simulink model "c00007M_harness"  (R2018a)
settings: Solver=ode3  StartTime=0.0  StopTime=10.0  RelTol=1e-3  EnableMultiTasking=on
undefined symbols (not defined in the file): b, DiscIntNeverNeededParam, J, K, L, PosMinimaW3, PosMinimaW4, R, sigbuilder_block
(part 6 of 74)

== system c00007M_harness/Eval92 ==
  In1 : Inport
  In2 : Inport  Port=2
  In3 : Inport  Port=3
  In4 : Inport  Port=4
  Data Type Conversion{,1..3} (4 alike) : DataTypeConversion
  Memory{1..4} (4 alike) : Memory  InitialCondition=1
  MinMax : MinMax  Inputs=4
  MinMax{1..4} (4 alike) : MinMax  Inputs=2
  ROOut{1..4} (4 alike) : RelationalOperator  Operator===  OutDataTypeStr=boolean  RndMeth=Simplest
  Out1 : Outport
  wires:
  Data Type Conversion3/1 -> MinMax4/1
  Data Type Conversion2/1 -> MinMax3/1
  Data Type Conversion1/1 -> MinMax2/1
  Data Type Conversion/1 -> MinMax1/1
  MinMax1/1 -> Memory1/1, MinMax/1
  ROOut4/1 -> Data Type Conversion3/1
  MinMax2/1 -> Memory2/1, MinMax/2
  ROOut1/1 -> Data Type Conversion/1
  Memory2/1 -> MinMax2/2
  Memory4/1 -> MinMax4/2
  Memory3/1 -> MinMax3/2
  ROOut2/1 -> Data Type Conversion1/1
  ROOut3/1 -> Data Type Conversion2/1
  MinMax3/1 -> Memory3/1, MinMax/3
  MinMax4/1 -> Memory4/1, MinMax/4
  Memory1/1 -> MinMax1/2
  [out4] -> ROOut4/2
  In4/1 -> ROOut4/1
  [out2] -> ROOut2/2
  In1/1 -> ROOut1/1
  In2/1 -> ROOut2/1
  [out1] -> ROOut1/2
  In3/1 -> ROOut3/1
  [out3] -> ROOut3/2
  MinMax/1 -> Out1/1

== system c00007M_harness/Eval93 ==
  In1 : Inport
  In2 : Inport  Port=2
  In3 : Inport  Port=3
  In4 : Inport  Port=4
  Data Type Conversion{,1..3} (4 alike) : DataTypeConversion
  Memory{1..4} (4 alike) : Memory  InitialCondition=1
  MinMax : MinMax  Inputs=4
  MinMax{1..4} (4 alike) : MinMax  Inputs=2
  ROOut{1..4} (4 alike) : RelationalOperator  Operator===  OutDataTypeStr=boolean  RndMeth=Simplest
  Out1 : Outport
  wires:
  Data Type Conversion3/1 -> MinMax4/1
  Data Type Conversion2/1 -> MinMax3/1
  Data Type Conversion1/1 -> MinMax2/1
  Data Type Conversion/1 -> MinMax1/1
  MinMax1/1 -> Memory1/1, MinMax/1
  ROOut4/1 -> Data Type Conversion3/1
  MinMax2/1 -> Memory2/1, MinMax/2
  ROOut1/1 -> Data Type Conversion/1
  Memory2/1 -> MinMax2/2
  Memory4/1 -> MinMax4/2
  Memory3/1 -> MinMax3/2
  ROOut2/1 -> Data Type Conversion1/1
  ROOut3/1 -> Data Type Conversion2/1
  MinMax3/1 -> Memory3/1, MinMax/3
  MinMax4/1 -> Memory4/1, MinMax/4
  Memory1/1 -> MinMax1/2
  [out4] -> ROOut4/2
  In4/1 -> ROOut4/1
  [out2] -> ROOut2/2
  In1/1 -> ROOut1/1
  In2/1 -> ROOut2/1
  [out1] -> ROOut1/2
  In3/1 -> ROOut3/1
  [out3] -> ROOut3/2
  MinMax/1 -> Out1/1

== system c00007M_harness/Eval94 ==
  In1 : Inport
  In2 : Inport  Port=2
  In3 : Inport  Port=3
  In4 : Inport  Port=4
  Data Type Conversion{,1..3} (4 alike) : DataTypeConversion
  Memory{1..4} (4 alike) : Memory  InitialCondition=1
  MinMax : MinMax  Inputs=4
  MinMax{1..4} (4 alike) : MinMax  Inputs=2
  ROOut{1..4} (4 alike) : RelationalOperator  Operator===  OutDataTypeStr=boolean  RndMeth=Simplest
  Out1 : Outport
  wires:
  Data Type Conversion3/1 -> MinMax4/1
  Data Type Conversion2/1 -> MinMax3/1
  Data Type Conversion1/1 -> MinMax2/1
  Data Type Conversion/1 -> MinMax1/1
  MinMax1/1 -> Memory1/1, MinMax/1
  ROOut4/1 -> Data Type Conversion3/1
  MinMax2/1 -> Memory2/1, MinMax/2
  ROOut1/1 -> Data Type Conversion/1
  Memory2/1 -> MinMax2/2
  Memory4/1 -> MinMax4/2
  Memory3/1 -> MinMax3/2
  ROOut2/1 -> Data Type Conversion1/1
  ROOut3/1 -> Data Type Conversion2/1
  MinMax3/1 -> Memory3/1, MinMax/3
  MinMax4/1 -> Memory4/1, MinMax/4
  Memory1/1 -> MinMax1/2
  [out4] -> ROOut4/2
  In4/1 -> ROOut4/1
  [out2] -> ROOut2/2
  In1/1 -> ROOut1/1
  In2/1 -> ROOut2/1
  [out1] -> ROOut1/2
  In3/1 -> ROOut3/1
  [out3] -> ROOut3/2
  MinMax/1 -> Out1/1

== system c00007M_harness/Eval95 ==
  In1 : Inport
  In2 : Inport  Port=2
  In3 : Inport  Port=3
  In4 : Inport  Port=4
  Data Type Conversion{,1..3} (4 alike) : DataTypeConversion
  Memory{1..4} (4 alike) : Memory  InitialCondition=1
  MinMax : MinMax  Inputs=4
  MinMax{1..4} (4 alike) : MinMax  Inputs=2
  ROOut{1..4} (4 alike) : RelationalOperator  Operator===  OutDataTypeStr=boolean  RndMeth=Simplest
  Out1 : Outport
  wires:
  Data Type Conversion3/1 -> MinMax4/1
  Data Type Conversion2/1 -> MinMax3/1
  Data Type Conversion1/1 -> MinMax2/1
  Data Type Conversion/1 -> MinMax1/1
  MinMax1/1 -> Memory1/1, MinMax/1
  ROOut4/1 -> Data Type Conversion3/1
  MinMax2/1 -> Memory2/1, MinMax/2
  ROOut1/1 -> Data Type Conversion/1
  Memory2/1 -> MinMax2/2
  Memory4/1 -> MinMax4/2
  Memory3/1 -> MinMax3/2
  ROOut2/1 -> Data Type Conversion1/1
  ROOut3/1 -> Data Type Conversion2/1
  MinMax3/1 -> Memory3/1, MinMax/3
  MinMax4/1 -> Memory4/1, MinMax/4
  Memory1/1 -> MinMax1/2
  [out4] -> ROOut4/2
  In4/1 -> ROOut4/1
  [out2] -> ROOut2/2
  In1/1 -> ROOut1/1
  In2/1 -> ROOut2/1
  [out1] -> ROOut1/2
  In3/1 -> ROOut3/1
  [out3] -> ROOut3/2
  MinMax/1 -> Out1/1

== system c00007M_harness/Eval96 ==
  In1 : Inport
  In2 : Inport  Port=2
  In3 : Inport  Port=3
  In4 : Inport  Port=4
  Data Type Conversion{,1..3} (4 alike) : DataTypeConversion
  Memory{1..4} (4 alike) : Memory  InitialCondition=1
  MinMax : MinMax  Inputs=4
  MinMax{1..4} (4 alike) : MinMax  Inputs=2
  ROOut{1..4} (4 alike) : RelationalOperator  Operator===  OutDataTypeStr=boolean  RndMeth=Simplest
  Out1 : Outport
  wires:
  Data Type Conversion3/1 -> MinMax4/1
  Data Type Conversion2/1 -> MinMax3/1
  Data Type Conversion1/1 -> MinMax2/1
  Data Type Conversion/1 -> MinMax1/1
  MinMax1/1 -> Memory1/1, MinMax/1
  ROOut4/1 -> Data Type Conversion3/1
  MinMax2/1 -> Memory2/1, MinMax/2
  ROOut1/1 -> Data Type Conversion/1
  Memory2/1 -> MinMax2/2
  Memory4/1 -> MinMax4/2
  Memory3/1 -> MinMax3/2
  ROOut2/1 -> Data Type Conversion1/1
  ROOut3/1 -> Data Type Conversion2/1
  MinMax3/1 -> Memory3/1, MinMax/3
  MinMax4/1 -> Memory4/1, MinMax/4
  Memory1/1 -> MinMax1/2
  [out4] -> ROOut4/2
  In4/1 -> ROOut4/1
  [out2] -> ROOut2/2
  In1/1 -> ROOut1/1
  In2/1 -> ROOut2/1
  [out1] -> ROOut1/2
  In3/1 -> ROOut3/1
  [out3] -> ROOut3/2
  MinMax/1 -> Out1/1

== system c00007M_harness/Eval97 ==
  In1 : Inport
  In2 : Inport  Port=2
  In3 : Inport  Port=3
  In4 : Inport  Port=4
  Data Type Conversion{,1..3} (4 alike) : DataTypeConversion
  Memory{1..4} (4 alike) : Memory  InitialCondition=1
  MinMax : MinMax  Inputs=4
  MinMax{1..4} (4 alike) : MinMax  Inputs=2
  ROOut{1..4} (4 alike) : RelationalOperator  Operator===  OutDataTypeStr=boolean  RndMeth=Simplest
  Out1 : Outport
  wires:
  Data Type Conversion3/1 -> MinMax4/1
  Data Type Conversion2/1 -> MinMax3/1
  Data Type Conversion1/1 -> MinMax2/1
  Data Type Conversion/1 -> MinMax1/1
  MinMax1/1 -> Memory1/1, MinMax/1
  ROOut4/1 -> Data Type Conversion3/1
  MinMax2/1 -> Memory2/1, MinMax/2
  ROOut1/1 -> Data Type Conversion/1
  Memory2/1 -> MinMax2/2
  Memory4/1 -> MinMax4/2
  Memory3/1 -> MinMax3/2
  ROOut2/1 -> Data Type Conversion1/1
  ROOut3/1 -> Data Type Conversion2/1
  MinMax3/1 -> Memory3/1, MinMax/3
  MinMax4/1 -> Memory4/1, MinMax/4
  Memory1/1 -> MinMax1/2
  [out4] -> ROOut4/2
  In4/1 -> ROOut4/1
  [out2] -> ROOut2/2
  In1/1 -> ROOut1/1
  In2/1 -> ROOut2/1
  [out1] -> ROOut1/2
  In3/1 -> ROOut3/1
  [out3] -> ROOut3/2
  MinMax/1 -> Out1/1

== system c00007M_harness/Eval98 ==
  In1 : Inport
  In2 : Inport  Port=2
  In3 : Inport  Port=3
  In4 : Inport  Port=4
  Data Type Conversion{,1..3} (4 alike) : DataTypeConversion
  Memory{1..4} (4 alike) : Memory  InitialCondition=1
  MinMax : MinMax  Inputs=4
  MinMax{1..4} (4 alike) : MinMax  Inputs=2
  ROOut{1..4} (4 alike) : RelationalOperator  Operator===  OutDataTypeStr=boolean  RndMeth=Simplest
  Out1 : Outport
  wires:
  Data Type Conversion3/1 -> MinMax4/1
  Data Type Conversion2/1 -> MinMax3/1
  Data Type Conversion1/1 -> MinMax2/1
  Data Type Conversion/1 -> MinMax1/1
  MinMax1/1 -> Memory1/1, MinMax/1
  ROOut4/1 -> Data Type Conversion3/1
  MinMax2/1 -> Memory2/1, MinMax/2
  ROOut1/1 -> Data Type Conversion/1
  Memory2/1 -> MinMax2/2
  Memory4/1 -> MinMax4/2
  Memory3/1 -> MinMax3/2
  ROOut2/1 -> Data Type Conversion1/1
  ROOut3/1 -> Data Type Conversion2/1
  MinMax3/1 -> Memory3/1, MinMax/3
  MinMax4/1 -> Memory4/1, MinMax/4
  Memory1/1 -> MinMax1/2
  [out4] -> ROOut4/2
  In4/1 -> ROOut4/1
  [out2] -> ROOut2/2
  In1/1 -> ROOut1/1
  In2/1 -> ROOut2/1
  [out1] -> ROOut1/2
  In3/1 -> ROOut3/1
  [out3] -> ROOut3/2
  MinMax/1 -> Out1/1

== system c00007M_harness/Eval99 ==
  In1 : Inport
  In2 : Inport  Port=2
  In3 : Inport  Port=3
  In4 : Inport  Port=4
  Data Type Conversion{,1..3} (4 alike) : DataTypeConversion
  Memory{1..4} (4 alike) : Memory  InitialCondition=1
  MinMax : MinMax  Inputs=4
  MinMax{1..4} (4 alike) : MinMax  Inputs=2
  ROOut{1..4} (4 alike) : RelationalOperator  Operator===  OutDataTypeStr=boolean  RndMeth=Simplest
  Out1 : Outport
  wires:
  Data Type Conversion3/1 -> MinMax4/1
  Data Type Conversion2/1 -> MinMax3/1
  Data Type Conversion1/1 -> MinMax2/1
  Data Type Conversion/1 -> MinMax1/1
  MinMax1/1 -> Memory1/1, MinMax/1
  ROOut4/1 -> Data Type Conversion3/1
  MinMax2/1 -> Memory2/1, MinMax/2
  ROOut1/1 -> Data Type Conversion/1
  Memory2/1 -> MinMax2/2
  Memory4/1 -> MinMax4/2
  Memory3/1 -> MinMax3/2
  ROOut2/1 -> Data Type Conversion1/1
  ROOut3/1 -> Data Type Conversion2/1
  MinMax3/1 -> Memory3/1, MinMax/3
  MinMax4/1 -> Memory4/1, MinMax/4
  Memory1/1 -> MinMax1/2
  [out4] -> ROOut4/2
  In4/1 -> ROOut4/1
  [out2] -> ROOut2/2
  In1/1 -> ROOut1/1
  In2/1 -> ROOut2/1
  [out1] -> ROOut1/2
  In3/1 -> ROOut3/1
  [out3] -> ROOut3/2
  MinMax/1 -> Out1/1

== system c00007M_harness/Inputs ==
  Demux : Demux  Tag=STV Demux  Outputs=14
  FromWs : FromWorkspace  Tag=STV FromWs  VariableName=tuvar  SampleTime=0
  DW1 : Outport  Tag=STV Outport
  DW2 : Outport  Tag=STV Outport  Port=2
  DW3 : Outport  Tag=STV Outport  Port=3
  P1W2 : Outport  Tag=STV Outport  Port=4
  P2W3 : Outport  Tag=STV Outport  Port=5
  P3W4 : Outport  Tag=STV Outport  Port=6
  O1 : Outport  Tag=STV Outport  Port=7
  O2 : Outport  Tag=STV Outport  Port=8
  O3 : Outport  Tag=STV Outport  Port=9
  O4 : Outport  Tag=STV Outport  Port=10
  LD : Outport  Tag=STV Outport  Port=11
  CW1C : Outport  Tag=STV Outport  Port=12
  CW2C : Outport  Tag=STV Outport  Port=13
  CW4C : Outport  Tag=STV Outport  Port=14
  wires:
  Demux/14 -> CW4C/1
  Demux/13 -> CW2C/1
  Demux/12 -> CW1C/1
  Demux/11 -> LD/1
  Demux/10 -> O4/1
  Demux/9 -> O3/1
  Demux/8 -> O2/1
  Demux/7 -> O1/1
  Demux/6 -> P3W4/1
  Demux/5 -> P2W3/1
  Demux/4 -> P1W2/1
  Demux/3 -> DW3/1
  Demux/2 -> DW2/1
  Demux/1 -> DW1/1
  FromWs/1 -> Demux/1

== system c00007M_harness/M001 ==
  DW1 : Inport  OutMin=0  OutMax=4  OutDataTypeStr=int8
  DW2 : Inport  Port=2  OutMin=0  OutMax=4  OutDataTypeStr=int8
  DW3 : Inport  Port=3  OutMin=0  OutMax=4  OutDataTypeStr=int8
  P1W2 : Inport  Port=4  OutMin=0  OutMax=4  OutDataTypeStr=int8
  P2W3 : Inport  Port=5  OutMin=0  OutMax=4  OutDataTypeStr=int8
  P3W4 : Inport  Port=6  OutMin=0  OutMax=4  OutDataTypeStr=int8
  O1 : Inport  Port=7  OutDataTypeStr=boolean
  O2 : Inport  Port=8  OutDataTypeStr=boolean
  O3 : Inport  Port=9  OutDataTypeStr=boolean
  O4 : Inport  Port=10  OutDataTypeStr=boolean
  LD : Inport  Port=11  OutDataTypeStr=boolean
  CW1C : Inport  Port=12  OutMin=0  OutMax=4  OutDataTypeStr=int8
  CW2C : Inport  Port=13  OutMin=0  OutMax=4  OutDataTypeStr=int8
  CW4C : Inport  Port=14  OutMin=0  OutMax=4  OutDataTypeStr=int8
  Cyber : Subsystem
  M{,1..3} (4 alike) : Memory
  Physical : Subsystem
  S1 : Subsystem
  S2 : Subsystem
  S3 : Subsystem
  S4 : Subsystem
  W1Pos : Outport
  W2Pos : Outport  Port=2
  W3Pos : Outport  Port=3
  W4Pos : Outport  Port=4
  wires:
  M3/1 -> Cyber/4(PosW4)
  P2W3/1 -> Cyber/9(P2W3)
  S1/1(SensorOut) -> M/1
  CW2C/1 -> Cyber/17(CW2C)
  CW4C/1 -> Cyber/18(CW4C)
  Physical/1(W1) -> W1Pos/1, S1/1(PhyMeasure)
  O4/1 -> Cyber/14(OW4)
  S3/1(SensorOut) -> M2/1
  O2/1 -> Cyber/12(OW2)
  Cyber/3(W3) -> Physical/3(InW3)
  LD/1 -> Cyber/15(LD)
  O1/1 -> Cyber/11(OW1)
  Cyber/1(W1) -> Physical/1(InW1)
  Cyber/2(W2) -> Physical/2(InW2)
  M2/1 -> Cyber/3(PosW3)
  P1W2/1 -> Cyber/8(P1W2)
  CW1C/1 -> Cyber/16(CW1C)
  O3/1 -> Cyber/13(OW3)
  DW3/1 -> Cyber/7(DW3)
  S4/1(SensorOut) -> M3/1
  M1/1 -> Cyber/2(PosW2)
  Physical/3(W3) -> W3Pos/1, S3/1(PhyMeasure)
  M/1 -> Cyber/1(PosW1)
  DW1/1 -> Cyber/5(DW1)
  Physical/2(W2) -> W2Pos/1, S2/1(PhyMeasure)
  S2/1(SensorOut) -> M1/1
  P3W4/1 -> Cyber/10(P3W4)
  DW2/1 -> Cyber/6(DW2)
  Physical/4(W4) -> W4Pos/1, S4/1(PhyMeasure)
  Cyber/4(W4) -> Physical/4(InW4)

== system c00007M_harness/M002 ==
  DW1 : Inport  OutMin=0  OutMax=4  OutDataTypeStr=int8
  DW2 : Inport  Port=2  OutMin=0  OutMax=4  OutDataTypeStr=int8
  DW3 : Inport  Port=3  OutMin=0  OutMax=4  OutDataTypeStr=int8
  P1W2 : Inport  Port=4  OutMin=0  OutMax=4  OutDataTypeStr=int8
  P2W3 : Inport  Port=5  OutMin=0  OutMax=4  OutDataTypeStr=int8
  P3W4 : Inport  Port=6  OutMin=0  OutMax=4  OutDataTypeStr=int8
  O1 : Inport  Port=7  OutDataTypeStr=boolean
  O2 : Inport  Port=8  OutDataTypeStr=boolean
  O3 : Inport  Port=9  OutDataTypeStr=boolean
  O4 : Inport  Port=10  OutDataTypeStr=boolean
  LD : Inport  Port=11  OutDataTypeStr=boolean
  CW1C : Inport  Port=12  OutMin=0  OutMax=4  OutDataTypeStr=int8
  CW2C : Inport  Port=13  OutMin=0  OutMax=4  OutDataTypeStr=int8
  CW4C : Inport  Port=14  OutMin=0  OutMax=4  OutDataTypeStr=int8
  Cyber : Subsystem
  M{,1..3} (4 alike) : Memory
  Physical : Subsystem
  S1 : Subsystem
  S2 : Subsystem
  S3 : Subsystem
  S4 : Subsystem
  W1Pos : Outport
  W2Pos : Outport  Port=2
  W3Pos : Outport  Port=3
  W4Pos : Outport  Port=4
  wires:
  Cyber/4(W4) -> Physical/4(InW4)
  Physical/4(W4) -> S4/1(PhyMeasure), W4Pos/1
  DW2/1 -> Cyber/6(DW2)
  P3W4/1 -> Cyber/10(P3W4)
  S2/1(SensorOut) -> M1/1
  Physical/2(W2) -> S2/1(PhyMeasure), W2Pos/1
  DW1/1 -> Cyber/5(DW1)
  M/1 -> Cyber/1(PosW1)
  Physical/3(W3) -> S3/1(PhyMeasure), W3Pos/1
  M1/1 -> Cyber/2(PosW2)
  S4/1(SensorOut) -> M3/1
  DW3/1 -> Cyber/7(DW3)
  O3/1 -> Cyber/13(OW3)
  CW1C/1 -> Cyber/16(CW1C)
  P1W2/1 -> Cyber/8(P1W2)
  M2/1 -> Cyber/3(PosW3)
  Cyber/2(W2) -> Physical/2(InW2)
  Cyber/1(W1) -> Physical/1(InW1)
  O1/1 -> Cyber/11(OW1)
  LD/1 -> Cyber/15(LD)
  Cyber/3(W3) -> Physical/3(InW3)
  O2/1 -> Cyber/12(OW2)
  S3/1(SensorOut) -> M2/1
  O4/1 -> Cyber/14(OW4)
  Physical/1(W1) -> S1/1(PhyMeasure), W1Pos/1
  CW4C/1 -> Cyber/18(CW4C)
  CW2C/1 -> Cyber/17(CW2C)
  S1/1(SensorOut) -> M/1
  P2W3/1 -> Cyber/9(P2W3)
  M3/1 -> Cyber/4(PosW4)

== system c00007M_harness/M003 ==
  DW1 : Inport  OutMin=0  OutMax=4  OutDataTypeStr=int8
  DW2 : Inport  Port=2  OutMin=0  OutMax=4  OutDataTypeStr=int8
  DW3 : Inport  Port=3  OutMin=0  OutMax=4  OutDataTypeStr=int8
  P1W2 : Inport  Port=4  OutMin=0  OutMax=4  OutDataTypeStr=int8
  P2W3 : Inport  Port=5  OutMin=0  OutMax=4  OutDataTypeStr=int8
  P3W4 : Inport  Port=6  OutMin=0  OutMax=4  OutDataTypeStr=int8
  O1 : Inport  Port=7  OutDataTypeStr=boolean
  O2 : Inport  Port=8  OutDataTypeStr=boolean
  O3 : Inport  Port=9  OutDataTypeStr=boolean
  O4 : Inport  Port=10  OutDataTypeStr=boolean
  LD : Inport  Port=11  OutDataTypeStr=boolean
  CW1C : Inport  Port=12  OutMin=0  OutMax=4  OutDataTypeStr=int8
  CW2C : Inport  Port=13  OutMin=0  OutMax=4  OutDataTypeStr=int8
  CW4C : Inport  Port=14  OutMin=0  OutMax=4  OutDataTypeStr=int8
  Cyber : Subsystem
  M{,1..3} (4 alike) : Memory
  Physical : Subsystem
  S1 : Subsystem
  S2 : Subsystem
  S3 : Subsystem
  S4 : Subsystem
  W1Pos : Outport
  W2Pos : Outport  Port=2
  W3Pos : Outport  Port=3
  W4Pos : Outport  Port=4
  wires:
  Cyber/4(W4) -> Physical/4(InW4)
  Physical/4(W4) -> S4/1(PhyMeasure), W4Pos/1
  DW2/1 -> Cyber/6(DW2)
  P3W4/1 -> Cyber/10(P3W4)
  S2/1(SensorOut) -> M1/1
  Physical/2(W2) -> S2/1(PhyMeasure), W2Pos/1
  DW1/1 -> Cyber/5(DW1)
  M/1 -> Cyber/1(PosW1)
  Physical/3(W3) -> S3/1(PhyMeasure), W3Pos/1
  M1/1 -> Cyber/2(PosW2)
  S4/1(SensorOut) -> M3/1
  DW3/1 -> Cyber/7(DW3)
  O3/1 -> Cyber/13(OW3)
  CW1C/1 -> Cyber/16(CW1C)
  P1W2/1 -> Cyber/8(P1W2)
  M2/1 -> Cyber/3(PosW3)
  Cyber/2(W2) -> Physical/2(InW2)
  Cyber/1(W1) -> Physical/1(InW1)
  O1/1 -> Cyber/11(OW1)
  LD/1 -> Cyber/15(LD)
  Cyber/3(W3) -> Physical/3(InW3)
  O2/1 -> Cyber/12(OW2)
  S3/1(SensorOut) -> M2/1
  O4/1 -> Cyber/14(OW4)
  Physical/1(W1) -> S1/1(PhyMeasure), W1Pos/1
  CW4C/1 -> Cyber/18(CW4C)
  CW2C/1 -> Cyber/17(CW2C)
  S1/1(SensorOut) -> M/1
  P2W3/1 -> Cyber/9(P2W3)
  M3/1 -> Cyber/4(PosW4)

== system c00007M_harness/M004 ==
  DW1 : Inport  OutMin=0  OutMax=4  OutDataTypeStr=int8
  DW2 : Inport  Port=2  OutMin=0  OutMax=4  OutDataTypeStr=int8
  DW3 : Inport  Port=3  OutMin=0  OutMax=4  OutDataTypeStr=int8
  P1W2 : Inport  Port=4  OutMin=0  OutMax=4  OutDataTypeStr=int8
  P2W3 : Inport  Port=5  OutMin=0  OutMax=4  OutDataTypeStr=int8
  P3W4 : Inport  Port=6  OutMin=0  OutMax=4  OutDataTypeStr=int8
  O1 : Inport  Port=7  OutDataTypeStr=boolean
  O2 : Inport  Port=8  OutDataTypeStr=boolean
  O3 : Inport  Port=9  OutDataTypeStr=boolean
  O4 : Inport  Port=10  OutDataTypeStr=boolean
  LD : Inport  Port=11  OutDataTypeStr=boolean
  CW1C : Inport  Port=12  OutMin=0  OutMax=4  OutDataTypeStr=int8
  CW2C : Inport  Port=13  OutMin=0  OutMax=4  OutDataTypeStr=int8
  CW4C : Inport  Port=14  OutMin=0  OutMax=4  OutDataTypeStr=int8
  Cyber : Subsystem
  M{,1..3} (4 alike) : Memory
  Physical : Subsystem
  S1 : Subsystem
  S2 : Subsystem
  S3 : Subsystem
  S4 : Subsystem
  W1Pos : Outport
  W2Pos : Outport  Port=2
  W3Pos : Outport  Port=3
  W4Pos : Outport  Port=4
  wires:
  Cyber/4(W4) -> Physical/4(InW4)
  Physical/4(W4) -> S4/1(PhyMeasure), W4Pos/1
  DW2/1 -> Cyber/6(DW2)
  P3W4/1 -> Cyber/10(P3W4)
  S2/1(SensorOut) -> M1/1
  Physical/2(W2) -> S2/1(PhyMeasure), W2Pos/1
  DW1/1 -> Cyber/5(DW1)
  M/1 -> Cyber/1(PosW1)
  Physical/3(W3) -> S3/1(PhyMeasure), W3Pos/1
  M1/1 -> Cyber/2(PosW2)
  S4/1(SensorOut) -> M3/1
  DW3/1 -> Cyber/7(DW3)
  O3/1 -> Cyber/13(OW3)
  CW1C/1 -> Cyber/16(CW1C)
  P1W2/1 -> Cyber/8(P1W2)
  M2/1 -> Cyber/3(PosW3)
  Cyber/2(W2) -> Physical/2(InW2)
  Cyber/1(W1) -> Physical/1(InW1)
  O1/1 -> Cyber/11(OW1)
  LD/1 -> Cyber/15(LD)
  Cyber/3(W3) -> Physical/3(InW3)
  O2/1 -> Cyber/12(OW2)
  S3/1(SensorOut) -> M2/1
  O4/1 -> Cyber/14(OW4)
  Physical/1(W1) -> S1/1(PhyMeasure), W1Pos/1
  CW4C/1 -> Cyber/18(CW4C)
  CW2C/1 -> Cyber/17(CW2C)
  S1/1(SensorOut) -> M/1
  P2W3/1 -> Cyber/9(P2W3)
  M3/1 -> Cyber/4(PosW4)

== system c00007M_harness/M005 ==
  DW1 : Inport  OutMin=0  OutMax=4  OutDataTypeStr=int8
  DW2 : Inport  Port=2  OutMin=0  OutMax=4  OutDataTypeStr=int8
  DW3 : Inport  Port=3  OutMin=0  OutMax=4  OutDataTypeStr=int8
  P1W2 : Inport  Port=4  OutMin=0  OutMax=4  OutDataTypeStr=int8
  P2W3 : Inport  Port=5  OutMin=0  OutMax=4  OutDataTypeStr=int8
  P3W4 : Inport  Port=6  OutMin=0  OutMax=4  OutDataTypeStr=int8
  O1 : Inport  Port=7  OutDataTypeStr=boolean
  O2 : Inport  Port=8  OutDataTypeStr=boolean
  O3 : Inport  Port=9  OutDataTypeStr=boolean
  O4 : Inport  Port=10  OutDataTypeStr=boolean
  LD : Inport  Port=11  OutDataTypeStr=boolean
  CW1C : Inport  Port=12  OutMin=0  OutMax=4  OutDataTypeStr=int8
  CW2C : Inport  Port=13  OutMin=0  OutMax=4  OutDataTypeStr=int8
  CW4C : Inport  Port=14  OutMin=0  OutMax=4  OutDataTypeStr=int8
  Cyber : Subsystem
  M{,1..3} (4 alike) : Memory
  Physical : Subsystem
  S1 : Subsystem
  S2 : Subsystem
  S3 : Subsystem
  S4 : Subsystem
  W1Pos : Outport
  W2Pos : Outport  Port=2
  W3Pos : Outport  Port=3
  W4Pos : Outport  Port=4
  wires:
  Cyber/4(W4) -> Physical/4(InW4)
  Physical/4(W4) -> S4/1(PhyMeasure), W4Pos/1
  DW2/1 -> Cyber/6(DW2)
  P3W4/1 -> Cyber/10(P3W4)
  S2/1(SensorOut) -> M1/1
  Physical/2(W2) -> S2/1(PhyMeasure), W2Pos/1
  DW1/1 -> Cyber/5(DW1)
  M/1 -> Cyber/1(PosW1)
  Physical/3(W3) -> S3/1(PhyMeasure), W3Pos/1
  M1/1 -> Cyber/2(PosW2)
  S4/1(SensorOut) -> M3/1
  DW3/1 -> Cyber/7(DW3)
  O3/1 -> Cyber/13(OW3)
  CW1C/1 -> Cyber/16(CW1C)
  P1W2/1 -> Cyber/8(P1W2)
  M2/1 -> Cyber/3(PosW3)
  Cyber/2(W2) -> Physical/2(InW2)
  Cyber/1(W1) -> Physical/1(InW1)
  O1/1 -> Cyber/11(OW1)
  LD/1 -> Cyber/15(LD)
  Cyber/3(W3) -> Physical/3(InW3)
  O2/1 -> Cyber/12(OW2)
  S3/1(SensorOut) -> M2/1
  O4/1 -> Cyber/14(OW4)
  Physical/1(W1) -> S1/1(PhyMeasure), W1Pos/1
  CW4C/1 -> Cyber/18(CW4C)
  CW2C/1 -> Cyber/17(CW2C)
  S1/1(SensorOut) -> M/1
  P2W3/1 -> Cyber/9(P2W3)
  M3/1 -> Cyber/4(PosW4)

== system c00007M_harness/M006 ==
  DW1 : Inport  OutMin=0  OutMax=4  OutDataTypeStr=int8
  DW2 : Inport  Port=2  OutMin=0  OutMax=4  OutDataTypeStr=int8
  DW3 : Inport  Port=3  OutMin=0  OutMax=4  OutDataTypeStr=int8
  P1W2 : Inport  Port=4  OutMin=0  OutMax=4  OutDataTypeStr=int8
  P2W3 : Inport  Port=5  OutMin=0  OutMax=4  OutDataTypeStr=int8
  P3W4 : Inport  Port=6  OutMin=0  OutMax=4  OutDataTypeStr=int8
  O1 : Inport  Port=7  OutDataTypeStr=boolean
  O2 : Inport  Port=8  OutDataTypeStr=boolean
  O3 : Inport  Port=9  OutDataTypeStr=boolean
  O4 : Inport  Port=10  OutDataTypeStr=boolean
  LD : Inport  Port=11  OutDataTypeStr=boolean
  CW1C : Inport  Port=12  OutMin=0  OutMax=4  OutDataTypeStr=int8
  CW2C : Inport  Port=13  OutMin=0  OutMax=4  OutDataTypeStr=int8
  CW4C : Inport  Port=14  OutMin=0  OutMax=4  OutDataTypeStr=int8
  Cyber : Subsystem
  M{,1..3} (4 alike) : Memory
  Physical : Subsystem
  S1 : Subsystem
  S2 : Subsystem
  S3 : Subsystem
  S4 : Subsystem
  W1Pos : Outport
  W2Pos : Outport  Port=2
  W3Pos : Outport  Port=3
  W4Pos : Outport  Port=4
  wires:
  Cyber/4(W4) -> Physical/4(InW4)
  Physical/4(W4) -> S4/1(PhyMeasure), W4Pos/1
  DW2/1 -> Cyber/6(DW2)
  P3W4/1 -> Cyber/10(P3W4)
  S2/1(SensorOut) -> M1/1
  Physical/2(W2) -> S2/1(PhyMeasure), W2Pos/1
  DW1/1 -> Cyber/5(DW1)
  M/1 -> Cyber/1(PosW1)
  Physical/3(W3) -> S3/1(PhyMeasure), W3Pos/1
  M1/1 -> Cyber/2(PosW2)
  S4/1(SensorOut) -> M3/1
  DW3/1 -> Cyber/7(DW3)
  O3/1 -> Cyber/13(OW3)
  CW1C/1 -> Cyber/16(CW1C)
  P1W2/1 -> Cyber/8(P1W2)
  M2/1 -> Cyber/3(PosW3)
  Cyber/2(W2) -> Physical/2(InW2)
  Cyber/1(W1) -> Physical/1(InW1)
  O1/1 -> Cyber/11(OW1)
  LD/1 -> Cyber/15(LD)
  Cyber/3(W3) -> Physical/3(InW3)
  O2/1 -> Cyber/12(OW2)
  S3/1(SensorOut) -> M2/1
  O4/1 -> Cyber/14(OW4)
  Physical/1(W1) -> S1/1(PhyMeasure), W1Pos/1
  CW4C/1 -> Cyber/18(CW4C)
  CW2C/1 -> Cyber/17(CW2C)
  S1/1(SensorOut) -> M/1
  P2W3/1 -> Cyber/9(P2W3)
  M3/1 -> Cyber/4(PosW4)

== system c00007M_harness/M007 ==
  DW1 : Inport  OutMin=0  OutMax=4  OutDataTypeStr=int8
  DW2 : Inport  Port=2  OutMin=0  OutMax=4  OutDataTypeStr=int8
  DW3 : Inport  Port=3  OutMin=0  OutMax=4  OutDataTypeStr=int8
  P1W2 : Inport  Port=4  OutMin=0  OutMax=4  OutDataTypeStr=int8
  P2W3 : Inport  Port=5  OutMin=0  OutMax=4  OutDataTypeStr=int8
  P3W4 : Inport  Port=6  OutMin=0  OutMax=4  OutDataTypeStr=int8
  O1 : Inport  Port=7  OutDataTypeStr=boolean
  O2 : Inport  Port=8  OutDataTypeStr=boolean
  O3 : Inport  Port=9  OutDataTypeStr=boolean
  O4 : Inport  Port=10  OutDataTypeStr=boolean
  LD : Inport  Port=11  OutDataTypeStr=boolean
  CW1C : Inport  Port=12  OutMin=0  OutMax=4  OutDataTypeStr=int8
  CW2C : Inport  Port=13  OutMin=0  OutMax=4  OutDataTypeStr=int8
  CW4C : Inport  Port=14  OutMin=0  OutMax=4  OutDataTypeStr=int8
  Cyber : Subsystem
  M{,1..3} (4 alike) : Memory
  Physical : Subsystem
  S1 : Subsystem
  S2 : Subsystem
  S3 : Subsystem
  S4 : Subsystem
  W1Pos : Outport
  W2Pos : Outport  Port=2
  W3Pos : Outport  Port=3
  W4Pos : Outport  Port=4
  wires:
  Cyber/4(W4) -> Physical/4(InW4)
  Physical/4(W4) -> S4/1(PhyMeasure), W4Pos/1
  DW2/1 -> Cyber/6(DW2)
  P3W4/1 -> Cyber/10(P3W4)
  S2/1(SensorOut) -> M1/1
  Physical/2(W2) -> S2/1(PhyMeasure), W2Pos/1
  DW1/1 -> Cyber/5(DW1)
  M/1 -> Cyber/1(PosW1)
  Physical/3(W3) -> S3/1(PhyMeasure), W3Pos/1
  M1/1 -> Cyber/2(PosW2)
  S4/1(SensorOut) -> M3/1
  DW3/1 -> Cyber/7(DW3)
  O3/1 -> Cyber/13(OW3)
  CW1C/1 -> Cyber/16(CW1C)
  P1W2/1 -> Cyber/8(P1W2)
  M2/1 -> Cyber/3(PosW3)
  Cyber/2(W2) -> Physical/2(InW2)
  Cyber/1(W1) -> Physical/1(InW1)
  O1/1 -> Cyber/11(OW1)
  LD/1 -> Cyber/15(LD)
  Cyber/3(W3) -> Physical/3(InW3)
  O2/1 -> Cyber/12(OW2)
  S3/1(SensorOut) -> M2/1
  O4/1 -> Cyber/14(OW4)
  Physical/1(W1) -> S1/1(PhyMeasure), W1Pos/1
  CW4C/1 -> Cyber/18(CW4C)
  CW2C/1 -> Cyber/17(CW2C)
  S1/1(SensorOut) -> M/1
  P2W3/1 -> Cyber/9(P2W3)
  M3/1 -> Cyber/4(PosW4)

== system c00007M_harness/M008 ==
  DW1 : Inport  OutMin=0  OutMax=4  OutDataTypeStr=int8
  DW2 : Inport  Port=2  OutMin=0  OutMax=4  OutDataTypeStr=int8
  DW3 : Inport  Port=3  OutMin=0  OutMax=4  OutDataTypeStr=int8
  P1W2 : Inport  Port=4  OutMin=0  OutMax=4  OutDataTypeStr=int8
  P2W3 : Inport  Port=5  OutMin=0  OutMax=4  OutDataTypeStr=int8
  P3W4 : Inport  Port=6  OutMin=0  OutMax=4  OutDataTypeStr=int8
  O1 : Inport  Port=7  OutDataTypeStr=boolean
  O2 : Inport  Port=8  OutDataTypeStr=boolean
  O3 : Inport  Port=9  OutDataTypeStr=boolean
  O4 : Inport  Port=10  OutDataTypeStr=boolean
  LD : Inport  Port=11  OutDataTypeStr=boolean
  CW1C : Inport  Port=12  OutMin=0  OutMax=4  OutDataTypeStr=int8
  CW2C : Inport  Port=13  OutMin=0  OutMax=4  OutDataTypeStr=int8
  CW4C : Inport  Port=14  OutMin=0  OutMax=4  OutDataTypeStr=int8
  Cyber : Subsystem
  M{,1..3} (4 alike) : Memory
  Physical : Subsystem
  S1 : Subsystem
  S2 : Subsystem
  S3 : Subsystem
  S4 : Subsystem
  W1Pos : Outport
  W2Pos : Outport  Port=2
  W3Pos : Outport  Port=3
  W4Pos : Outport  Port=4
  wires:
  Cyber/4(W4) -> Physical/4(InW4)
  Physical/4(W4) -> S4/1(PhyMeasure), W4Pos/1
  DW2/1 -> Cyber/6(DW2)
  P3W4/1 -> Cyber/10(P3W4)
  S2/1(SensorOut) -> M1/1
  Physical/2(W2) -> S2/1(PhyMeasure), W2Pos/1
  DW1/1 -> Cyber/5(DW1)
  M/1 -> Cyber/1(PosW1)
  Physical/3(W3) -> S3/1(PhyMeasure), W3Pos/1
  M1/1 -> Cyber/2(PosW2)
  S4/1(SensorOut) -> M3/1
  DW3/1 -> Cyber/7(DW3)
  O3/1 -> Cyber/13(OW3)
  CW1C/1 -> Cyber/16(CW1C)
  P1W2/1 -> Cyber/8(P1W2)
  M2/1 -> Cyber/3(PosW3)
  Cyber/2(W2) -> Physical/2(InW2)
  Cyber/1(W1) -> Physical/1(InW1)
  O1/1 -> Cyber/11(OW1)
  LD/1 -> Cyber/15(LD)
  Cyber/3(W3) -> Physical/3(InW3)
  O2/1 -> Cyber/12(OW2)
  S3/1(SensorOut) -> M2/1
  O4/1 -> Cyber/14(OW4)
  Physical/1(W1) -> S1/1(PhyMeasure), W1Pos/1
  CW4C/1 -> Cyber/18(CW4C)
  CW2C/1 -> Cyber/17(CW2C)
  S1/1(SensorOut) -> M/1
  P2W3/1 -> Cyber/9(P2W3)
  M3/1 -> Cyber/4(PosW4)

== system c00007M_harness/M009 ==
  DW1 : Inport  OutMin=0  OutMax=4  OutDataTypeStr=int8
  DW2 : Inport  Port=2  OutMin=0  OutMax=4  OutDataTypeStr=int8
  DW3 : Inport  Port=3  OutMin=0  OutMax=4  OutDataTypeStr=int8
  P1W2 : Inport  Port=4  OutMin=0  OutMax=4  OutDataTypeStr=int8
  P2W3 : Inport  Port=5  OutMin=0  OutMax=4  OutDataTypeStr=int8
  P3W4 : Inport  Port=6  OutMin=0  OutMax=4  OutDataTypeStr=int8
  O1 : Inport  Port=7  OutDataTypeStr=boolean
  O2 : Inport  Port=8  OutDataTypeStr=boolean
  O3 : Inport  Port=9  OutDataTypeStr=boolean
  O4 : Inport  Port=10  OutDataTypeStr=boolean
  LD : Inport  Port=11  OutDataTypeStr=boolean
  CW1C : Inport  Port=12  OutMin=0  OutMax=4  OutDataTypeStr=int8
  CW2C : Inport  Port=13  OutMin=0  OutMax=4  OutDataTypeStr=int8
  CW4C : Inport  Port=14  OutMin=0  OutMax=4  OutDataTypeStr=int8
  Cyber : Subsystem
  M{,1..3} (4 alike) : Memory
  Physical : Subsystem
  S1 : Subsystem
  S2 : Subsystem
  S3 : Subsystem
  S4 : Subsystem
  W1Pos : Outport
  W2Pos : Outport  Port=2
  W3Pos : Outport  Port=3
  W4Pos : Outport  Port=4
  wires:
  Cyber/4(W4) -> Physical/4(InW4)
  Physical/4(W4) -> S4/1(PhyMeasure), W4Pos/1
  DW2/1 -> Cyber/6(DW2)
  P3W4/1 -> Cyber/10(P3W4)
  S2/1(SensorOut) -> M1/1
  Physical/2(W2) -> S2/1(PhyMeasure), W2Pos/1
  DW1/1 -> Cyber/5(DW1)
  M/1 -> Cyber/1(PosW1)
  Physical/3(W3) -> S3/1(PhyMeasure), W3Pos/1
  M1/1 -> Cyber/2(PosW2)
  S4/1(SensorOut) -> M3/1
  DW3/1 -> Cyber/7(DW3)
  O3/1 -> Cyber/13(OW3)
  CW1C/1 -> Cyber/16(CW1C)
  P1W2/1 -> Cyber/8(P1W2)
  M2/1 -> Cyber/3(PosW3)
  Cyber/2(W2) -> Physical/2(InW2)
  Cyber/1(W1) -> Physical/1(InW1)
  O1/1 -> Cyber/11(OW1)
  LD/1 -> Cyber/15(LD)
  Cyber/3(W3) -> Physical/3(InW3)
  O2/1 -> Cyber/12(OW2)
  S3/1(SensorOut) -> M2/1
  O4/1 -> Cyber/14(OW4)
  Physical/1(W1) -> S1/1(PhyMeasure), W1Pos/1
  CW4C/1 -> Cyber/18(CW4C)
  CW2C/1 -> Cyber/17(CW2C)
  S1/1(SensorOut) -> M/1
  P2W3/1 -> Cyber/9(P2W3)
  M3/1 -> Cyber/4(PosW4)

== system c00007M_harness/M010 ==
  DW1 : Inport  OutMin=0  OutMax=4  OutDataTypeStr=int8
  DW2 : Inport  Port=2  OutMin=0  OutMax=4  OutDataTypeStr=int8
  DW3 : Inport  Port=3  OutMin=0  OutMax=4  OutDataTypeStr=int8
  P1W2 : Inport  Port=4  OutMin=0  OutMax=4  OutDataTypeStr=int8
  P2W3 : Inport  Port=5  OutMin=0  OutMax=4  OutDataTypeStr=int8
  P3W4 : Inport  Port=6  OutMin=0  OutMax=4  OutDataTypeStr=int8
  O1 : Inport  Port=7  OutDataTypeStr=boolean
  O2 : Inport  Port=8  OutDataTypeStr=boolean
  O3 : Inport  Port=9  OutDataTypeStr=boolean
  O4 : Inport  Port=10  OutDataTypeStr=boolean
  LD : Inport  Port=11  OutDataTypeStr=boolean
  CW1C : Inport  Port=12  OutMin=0  OutMax=4  OutDataTypeStr=int8
  CW2C : Inport  Port=13  OutMin=0  OutMax=4  OutDataTypeStr=int8
  CW4C : Inport  Port=14  OutMin=0  OutMax=4  OutDataTypeStr=int8
  Cyber : Subsystem
  M{,1..3} (4 alike) : Memory
  Physical : Subsystem
  S1 : Subsystem
  S2 : Subsystem
  S3 : Subsystem
  S4 : Subsystem
  W1Pos : Outport
  W2Pos : Outport  Port=2
  W3Pos : Outport  Port=3
  W4Pos : Outport  Port=4
  wires:
  Cyber/4(W4) -> Physical/4(InW4)
  Physical/4(W4) -> S4/1(PhyMeasure), W4Pos/1
  DW2/1 -> Cyber/6(DW2)
  P3W4/1 -> Cyber/10(P3W4)
  S2/1(SensorOut) -> M1/1
  Physical/2(W2) -> S2/1(PhyMeasure), W2Pos/1
  DW1/1 -> Cyber/5(DW1)
  M/1 -> Cyber/1(PosW1)
  Physical/3(W3) -> S3/1(PhyMeasure), W3Pos/1
  M1/1 -> Cyber/2(PosW2)
  S4/1(SensorOut) -> M3/1
  DW3/1 -> Cyber/7(DW3)
  O3/1 -> Cyber/13(OW3)
  CW1C/1 -> Cyber/16(CW1C)
  P1W2/1 -> Cyber/8(P1W2)
  M2/1 -> Cyber/3(PosW3)
  Cyber/2(W2) -> Physical/2(InW2)
  Cyber/1(W1) -> Physical/1(InW1)
  O1/1 -> Cyber/11(OW1)
  LD/1 -> Cyber/15(LD)
  Cyber/3(W3) -> Physical/3(InW3)
  O2/1 -> Cyber/12(OW2)
  S3/1(SensorOut) -> M2/1
  O4/1 -> Cyber/14(OW4)
  Physical/1(W1) -> S1/1(PhyMeasure), W1Pos/1
  CW4C/1 -> Cyber/18(CW4C)
  CW2C/1 -> Cyber/17(CW2C)
  S1/1(SensorOut) -> M/1
  P2W3/1 -> Cyber/9(P2W3)
  M3/1 -> Cyber/4(PosW4)

== system c00007M_harness/M011 ==
  DW1 : Inport  OutMin=0  OutMax=4  OutDataTypeStr=int8
  DW2 : Inport  Port=2  OutMin=0  OutMax=4  OutDataTypeStr=int8
  DW3 : Inport  Port=3  OutMin=0  OutMax=4  OutDataTypeStr=int8
  P1W2 : Inport  Port=4  OutMin=0  OutMax=4  OutDataTypeStr=int8
  P2W3 : Inport  Port=5  OutMin=0  OutMax=4  OutDataTypeStr=int8
  P3W4 : Inport  Port=6  OutMin=0  OutMax=4  OutDataTypeStr=int8
  O1 : Inport  Port=7  OutDataTypeStr=boolean
  O2 : Inport  Port=8  OutDataTypeStr=boolean
  O3 : Inport  Port=9  OutDataTypeStr=boolean
  O4 : Inport  Port=10  OutDataTypeStr=boolean
  LD : Inport  Port=11  OutDataTypeStr=boolean
  CW1C : Inport  Port=12  OutMin=0  OutMax=4  OutDataTypeStr=int8
  CW2C : Inport  Port=13  OutMin=0  OutMax=4  OutDataTypeStr=int8
  CW4C : Inport  Port=14  OutMin=0  OutMax=4  OutDataTypeStr=int8
  Cyber : Subsystem
  M{,1..3} (4 alike) : Memory
  Physical : Subsystem
  S1 : Subsystem
  S2 : Subsystem
  S3 : Subsystem
  S4 : Subsystem
  W1Pos : Outport
  W2Pos : Outport  Port=2
  W3Pos : Outport  Port=3
  W4Pos : Outport  Port=4
  wires:
  Cyber/4(W4) -> Physical/4(InW4)
  Physical/4(W4) -> S4/1(PhyMeasure), W4Pos/1
  DW2/1 -> Cyber/6(DW2)
  P3W4/1 -> Cyber/10(P3W4)
  S2/1(SensorOut) -> M1/1
  Physical/2(W2) -> S2/1(PhyMeasure), W2Pos/1
  DW1/1 -> Cyber/5(DW1)
  M/1 -> Cyber/1(PosW1)
  Physical/3(W3) -> S3/1(PhyMeasure), W3Pos/1
  M1/1 -> Cyber/2(PosW2)
  S4/1(SensorOut) -> M3/1
  DW3/1 -> Cyber/7(DW3)
  O3/1 -> Cyber/13(OW3)
  CW1C/1 -> Cyber/16(CW1C)
  P1W2/1 -> Cyber/8(P1W2)
  M2/1 -> Cyber/3(PosW3)
  Cyber/2(W2) -> Physical/2(InW2)
  Cyber/1(W1) -> Physical/1(InW1)
  O1/1 -> Cyber/11(OW1)
  LD/1 -> Cyber/15(LD)
  Cyber/3(W3) -> Physical/3(InW3)
  O2/1 -> Cyber/12(OW2)
  S3/1(SensorOut) -> M2/1
  O4/1 -> Cyber/14(OW4)
  Physical/1(W1) -> S1/1(PhyMeasure), W1Pos/1
  CW4C/1 -> Cyber/18(CW4C)
  CW2C/1 -> Cyber/17(CW2C)
  S1/1(SensorOut) -> M/1
  P2W3/1 -> Cyber/9(P2W3)
  M3/1 -> Cyber/4(PosW4)

== system c00007M_harness/M012 ==
  DW1 : Inport  OutMin=0  OutMax=4  OutDataTypeStr=int8
  DW2 : Inport  Port=2  OutMin=0  OutMax=4  OutDataTypeStr=int8
  DW3 : Inport  Port=3  OutMin=0  OutMax=4  OutDataTypeStr=int8
  P1W2 : Inport  Port=4  OutMin=0  OutMax=4  OutDataTypeStr=int8
  P2W3 : Inport  Port=5  OutMin=0  OutMax=4  OutDataTypeStr=int8
  P3W4 : Inport  Port=6  OutMin=0  OutMax=4  OutDataTypeStr=int8
  O1 : Inport  Port=7  OutDataTypeStr=boolean
  O2 : Inport  Port=8  OutDataTypeStr=boolean
  O3 : Inport  Port=9  OutDataTypeStr=boolean
  O4 : Inport  Port=10  OutDataTypeStr=boolean
  LD : Inport  Port=11  OutDataTypeStr=boolean
  CW1C : Inport  Port=12  OutMin=0  OutMax=4  OutDataTypeStr=int8
  CW2C : Inport  Port=13  OutMin=0  OutMax=4  OutDataTypeStr=int8
  CW4C : Inport  Port=14  OutMin=0  OutMax=4  OutDataTypeStr=int8
  Cyber : Subsystem
  M{,1..3} (4 alike) : Memory
  Physical : Subsystem
  S1 : Subsystem
  S2 : Subsystem
  S3 : Subsystem
  S4 : Subsystem
  W1Pos : Outport
  W2Pos : Outport  Port=2
  W3Pos : Outport  Port=3
  W4Pos : Outport  Port=4
  wires:
  Cyber/4(W4) -> Physical/4(InW4)
  Physical/4(W4) -> S4/1(PhyMeasure), W4Pos/1
  DW2/1 -> Cyber/6(DW2)
  P3W4/1 -> Cyber/10(P3W4)
  S2/1(SensorOut) -> M1/1
  Physical/2(W2) -> S2/1(PhyMeasure), W2Pos/1
  DW1/1 -> Cyber/5(DW1)
  M/1 -> Cyber/1(PosW1)
  Physical/3(W3) -> S3/1(PhyMeasure), W3Pos/1
  M1/1 -> Cyber/2(PosW2)
  S4/1(SensorOut) -> M3/1
  DW3/1 -> Cyber/7(DW3)
  O3/1 -> Cyber/13(OW3)
  CW1C/1 -> Cyber/16(CW1C)
  P1W2/1 -> Cyber/8(P1W2)
  M2/1 -> Cyber/3(PosW3)
  Cyber/2(W2) -> Physical/2(InW2)
  Cyber/1(W1) -> Physical/1(InW1)
  O1/1 -> Cyber/11(OW1)
  LD/1 -> Cyber/15(LD)
  Cyber/3(W3) -> Physical/3(InW3)
  O2/1 -> Cyber/12(OW2)
  S3/1(SensorOut) -> M2/1
  O4/1 -> Cyber/14(OW4)
  Physical/1(W1) -> S1/1(PhyMeasure), W1Pos/1
  CW4C/1 -> Cyber/18(CW4C)
  CW2C/1 -> Cyber/17(CW2C)
  S1/1(SensorOut) -> M/1
  P2W3/1 -> Cyber/9(P2W3)
  M3/1 -> Cyber/4(PosW4)

== system c00007M_harness/M013 ==
  DW1 : Inport  OutMin=0  OutMax=4  OutDataTypeStr=int8
  DW2 : Inport  Port=2  OutMin=0  OutMax=4  OutDataTypeStr=int8
  DW3 : Inport  Port=3  OutMin=0  OutMax=4  OutDataTypeStr=int8
  P1W2 : Inport  Port=4  OutMin=0  OutMax=4  OutDataTypeStr=int8
  P2W3 : Inport  Port=5  OutMin=0  OutMax=4  OutDataTypeStr=int8
  P3W4 : Inport  Port=6  OutMin=0  OutMax=4  OutDataTypeStr=int8
  O1 : Inport  Port=7  OutDataTypeStr=boolean
  O2 : Inport  Port=8  OutDataTypeStr=boolean
  O3 : Inport  Port=9  OutDataTypeStr=boolean
  O4 : Inport  Port=10  OutDataTypeStr=boolean
  LD : Inport  Port=11  OutDataTypeStr=boolean
  CW1C : Inport  Port=12  OutMin=0  OutMax=4  OutDataTypeStr=int8
  CW2C : Inport  Port=13  OutMin=0  OutMax=4  OutDataTypeStr=int8
  CW4C : Inport  Port=14  OutMin=0  OutMax=4  OutDataTypeStr=int8
  Cyber : Subsystem
  M{,1..3} (4 alike) : Memory
  Physical : Subsystem
  S1 : Subsystem
  S2 : Subsystem
  S3 : Subsystem
  S4 : Subsystem
  W1Pos : Outport
  W2Pos : Outport  Port=2
  W3Pos : Outport  Port=3
  W4Pos : Outport  Port=4
  wires:
  Cyber/4(W4) -> Physical/4(InW4)
  Physical/4(W4) -> S4/1(PhyMeasure), W4Pos/1
  DW2/1 -> Cyber/6(DW2)
  P3W4/1 -> Cyber/10(P3W4)
  S2/1(SensorOut) -> M1/1
  Physical/2(W2) -> S2/1(PhyMeasure), W2Pos/1
  DW1/1 -> Cyber/5(DW1)
  M/1 -> Cyber/1(PosW1)
  Physical/3(W3) -> S3/1(PhyMeasure), W3Pos/1
  M1/1 -> Cyber/2(PosW2)
  S4/1(SensorOut) -> M3/1
  DW3/1 -> Cyber/7(DW3)
  O3/1 -> Cyber/13(OW3)
  CW1C/1 -> Cyber/16(CW1C)
  P1W2/1 -> Cyber/8(P1W2)
  M2/1 -> Cyber/3(PosW3)
  Cyber/2(W2) -> Physical/2(InW2)
  Cyber/1(W1) -> Physical/1(InW1)
  O1/1 -> Cyber/11(OW1)
  LD/1 -> Cyber/15(LD)
  Cyber/3(W3) -> Physical/3(InW3)
  O2/1 -> Cyber/12(OW2)
  S3/1(SensorOut) -> M2/1
  O4/1 -> Cyber/14(OW4)
  Physical/1(W1) -> S1/1(PhyMeasure), W1Pos/1
  CW4C/1 -> Cyber/18(CW4C)
  CW2C/1 -> Cyber/17(CW2C)
  S1/1(SensorOut) -> M/1
  P2W3/1 -> Cyber/9(P2W3)
  M3/1 -> Cyber/4(PosW4)

== system c00007M_harness/M014 ==
  DW1 : Inport  OutMin=0  OutMax=4  OutDataTypeStr=int8
  DW2 : Inport  Port=2  OutMin=0  OutMax=4  OutDataTypeStr=int8
  DW3 : Inport  Port=3  OutMin=0  OutMax=4  OutDataTypeStr=int8
  P1W2 : Inport  Port=4  OutMin=0  OutMax=4  OutDataTypeStr=int8
  P2W3 : Inport  Port=5  OutMin=0  OutMax=4  OutDataTypeStr=int8
  P3W4 : Inport  Port=6  OutMin=0  OutMax=4  OutDataTypeStr=int8
  O1 : Inport  Port=7  OutDataTypeStr=boolean
  O2 : Inport  Port=8  OutDataTypeStr=boolean
  O3 : Inport  Port=9  OutDataTypeStr=boolean
  O4 : Inport  Port=10  OutDataTypeStr=boolean
  LD : Inport  Port=11  OutDataTypeStr=boolean
  CW1C : Inport  Port=12  OutMin=0  OutMax=4  OutDataTypeStr=int8
  CW2C : Inport  Port=13  OutMin=0  OutMax=4  OutDataTypeStr=int8
  CW4C : Inport  Port=14  OutMin=0  OutMax=4  OutDataTypeStr=int8
  Cyber : Subsystem
  M{,1..3} (4 alike) : Memory
  Physical : Subsystem
  S1 : Subsystem
  S2 : Subsystem
  S3 : Subsystem
  S4 : Subsystem
  W1Pos : Outport
  W2Pos : Outport  Port=2
  W3Pos : Outport  Port=3
  W4Pos : Outport  Port=4
  wires:
  Cyber/4(W4) -> Physical/4(InW4)
  Physical/4(W4) -> S4/1(PhyMeasure), W4Pos/1
  DW2/1 -> Cyber/6(DW2)
  P3W4/1 -> Cyber/10(P3W4)
  S2/1(SensorOut) -> M1/1
  Physical/2(W2) -> S2/1(PhyMeasure), W2Pos/1
  DW1/1 -> Cyber/5(DW1)
  M/1 -> Cyber/1(PosW1)
  Physical/3(W3) -> S3/1(PhyMeasure), W3Pos/1
  M1/1 -> Cyber/2(PosW2)
  S4/1(SensorOut) -> M3/1
  DW3/1 -> Cyber/7(DW3)
  O3/1 -> Cyber/13(OW3)
  CW1C/1 -> Cyber/16(CW1C)
  P1W2/1 -> Cyber/8(P1W2)
  M2/1 -> Cyber/3(PosW3)
  Cyber/2(W2) -> Physical/2(InW2)
  Cyber/1(W1) -> Physical/1(InW1)
  O1/1 -> Cyber/11(OW1)
  LD/1 -> Cyber/15(LD)
  Cyber/3(W3) -> Physical/3(InW3)
  O2/1 -> Cyber/12(OW2)
  S3/1(SensorOut) -> M2/1
  O4/1 -> Cyber/14(OW4)
  Physical/1(W1) -> S1/1(PhyMeasure), W1Pos/1
  CW4C/1 -> Cyber/18(CW4C)
  CW2C/1 -> Cyber/17(CW2C)
  S1/1(SensorOut) -> M/1
  P2W3/1 -> Cyber/9(P2W3)
  M3/1 -> Cyber/4(PosW4)

== system c00007M_harness/M015 ==
  DW1 : Inport  OutMin=0  OutMax=4  OutDataTypeStr=int8
  DW2 : Inport  Port=2  OutMin=0  OutMax=4  OutDataTypeStr=int8
  DW3 : Inport  Port=3  OutMin=0  OutMax=4  OutDataTypeStr=int8
  P1W2 : Inport  Port=4  OutMin=0  OutMax=4  OutDataTypeStr=int8
  P2W3 : Inport  Port=5  OutMin=0  OutMax=4  OutDataTypeStr=int8
  P3W4 : Inport  Port=6  OutMin=0  OutMax=4  OutDataTypeStr=int8
  O1 : Inport  Port=7  OutDataTypeStr=boolean
  O2 : Inport  Port=8  OutDataTypeStr=boolean
  O3 : Inport  Port=9  OutDataTypeStr=boolean
  O4 : Inport  Port=10  OutDataTypeStr=boolean
  LD : Inport  Port=11  OutDataTypeStr=boolean
  CW1C : Inport  Port=12  OutMin=0  OutMax=4  OutDataTypeStr=int8
  CW2C : Inport  Port=13  OutMin=0  OutMax=4  OutDataTypeStr=int8
  CW4C : Inport  Port=14  OutMin=0  OutMax=4  OutDataTypeStr=int8
  Cyber : Subsystem
  M{,1..3} (4 alike) : Memory
  Physical : Subsystem
  S1 : Subsystem
  S2 : Subsystem
  S3 : Subsystem
  S4 : Subsystem
  W1Pos : Outport
  W2Pos : Outport  Port=2
  W3Pos : Outport  Port=3
  W4Pos : Outport  Port=4
  wires:
  Cyber/4(W4) -> Physical/4(InW4)
  Physical/4(W4) -> S4/1(PhyMeasure), W4Pos/1
  DW2/1 -> Cyber/6(DW2)
  P3W4/1 -> Cyber/10(P3W4)
  S2/1(SensorOut) -> M1/1
  Physical/2(W2) -> S2/1(PhyMeasure), W2Pos/1
  DW1/1 -> Cyber/5(DW1)
  M/1 -> Cyber/1(PosW1)
  Physical/3(W3) -> S3/1(PhyMeasure), W3Pos/1
  M1/1 -> Cyber/2(PosW2)
  S4/1(SensorOut) -> M3/1
  DW3/1 -> Cyber/7(DW3)
  O3/1 -> Cyber/13(OW3)
  CW1C/1 -> Cyber/16(CW1C)
  P1W2/1 -> Cyber/8(P1W2)
  M2/1 -> Cyber/3(PosW3)
  Cyber/2(W2) -> Physical/2(InW2)
  Cyber/1(W1) -> Physical/1(InW1)
  O1/1 -> Cyber/11(OW1)
  LD/1 -> Cyber/15(LD)
  Cyber/3(W3) -> Physical/3(InW3)
  O2/1 -> Cyber/12(OW2)
  S3/1(SensorOut) -> M2/1
  O4/1 -> Cyber/14(OW4)
  Physical/1(W1) -> S1/1(PhyMeasure), W1Pos/1
  CW4C/1 -> Cyber/18(CW4C)
  CW2C/1 -> Cyber/17(CW2C)
  S1/1(SensorOut) -> M/1
  P2W3/1 -> Cyber/9(P2W3)
  M3/1 -> Cyber/4(PosW4)

== system c00007M_harness/M016 ==
  DW1 : Inport  OutMin=0  OutMax=4  OutDataTypeStr=int8
  DW2 : Inport  Port=2  OutMin=0  OutMax=4  OutDataTypeStr=int8
  DW3 : Inport  Port=3  OutMin=0  OutMax=4  OutDataTypeStr=int8
  P1W2 : Inport  Port=4  OutMin=0  OutMax=4  OutDataTypeStr=int8
  P2W3 : Inport  Port=5  OutMin=0  OutMax=4  OutDataTypeStr=int8
  P3W4 : Inport  Port=6  OutMin=0  OutMax=4  OutDataTypeStr=int8
  O1 : Inport  Port=7  OutDataTypeStr=boolean
  O2 : Inport  Port=8  OutDataTypeStr=boolean
  O3 : Inport  Port=9  OutDataTypeStr=boolean
  O4 : Inport  Port=10  OutDataTypeStr=boolean
  LD : Inport  Port=11  OutDataTypeStr=boolean
  CW1C : Inport  Port=12  OutMin=0  OutMax=4  OutDataTypeStr=int8
  CW2C : Inport  Port=13  OutMin=0  OutMax=4  OutDataTypeStr=int8
  CW4C : Inport  Port=14  OutMin=0  OutMax=4  OutDataTypeStr=int8
  Cyber : Subsystem
  M{,1..3} (4 alike) : Memory
  Physical : Subsystem
  S1 : Subsystem
  S2 : Subsystem
  S3 : Subsystem
  S4 : Subsystem
  W1Pos : Outport
  W2Pos : Outport  Port=2
  W3Pos : Outport  Port=3
  W4Pos : Outport  Port=4
  wires:
  Cyber/4(W4) -> Physical/4(InW4)
  Physical/4(W4) -> S4/1(PhyMeasure), W4Pos/1
  DW2/1 -> Cyber/6(DW2)
  P3W4/1 -> Cyber/10(P3W4)
  S2/1(SensorOut) -> M1/1
  Physical/2(W2) -> S2/1(PhyMeasure), W2Pos/1
  DW1/1 -> Cyber/5(DW1)
  M/1 -> Cyber/1(PosW1)
  Physical/3(W3) -> S3/1(PhyMeasure), W3Pos/1
  M1/1 -> Cyber/2(PosW2)
  S4/1(SensorOut) -> M3/1
  DW3/1 -> Cyber/7(DW3)
  O3/1 -> Cyber/13(OW3)
  CW1C/1 -> Cyber/16(CW1C)
  P1W2/1 -> Cyber/8(P1W2)
  M2/1 -> Cyber/3(PosW3)
  Cyber/2(W2) -> Physical/2(InW2)
  Cyber/1(W1) -> Physical/1(InW1)
  O1/1 -> Cyber/11(OW1)
  LD/1 -> Cyber/15(LD)
  Cyber/3(W3) -> Physical/3(InW3)
  O2/1 -> Cyber/12(OW2)
  S3/1(SensorOut) -> M2/1
  O4/1 -> Cyber/14(OW4)
  Physical/1(W1) -> S1/1(PhyMeasure), W1Pos/1
  CW4C/1 -> Cyber/18(CW4C)
  CW2C/1 -> Cyber/17(CW2C)
  S1/1(SensorOut) -> M/1
  P2W3/1 -> Cyber/9(P2W3)
  M3/1 -> Cyber/4(PosW4)

== system c00007M_harness/M017 ==
  DW1 : Inport  OutMin=0  OutMax=4  OutDataTypeStr=int8
  DW2 : Inport  Port=2  OutMin=0  OutMax=4  OutDataTypeStr=int8
  DW3 : Inport  Port=3  OutMin=0  OutMax=4  OutDataTypeStr=int8
  P1W2 : Inport  Port=4  OutMin=0  OutMax=4  OutDataTypeStr=int8
  P2W3 : Inport  Port=5  OutMin=0  OutMax=4  OutDataTypeStr=int8
  P3W4 : Inport  Port=6  OutMin=0  OutMax=4  OutDataTypeStr=int8
  O1 : Inport  Port=7  OutDataTypeStr=boolean
  O2 : Inport  Port=8  OutDataTypeStr=boolean
  O3 : Inport  Port=9  OutDataTypeStr=boolean
  O4 : Inport  Port=10  OutDataTypeStr=boolean
  LD : Inport  Port=11  OutDataTypeStr=boolean
  CW1C : Inport  Port=12  OutMin=0  OutMax=4  OutDataTypeStr=int8
  CW2C : Inport  Port=13  OutMin=0  OutMax=4  OutDataTypeStr=int8
  CW4C : Inport  Port=14  OutMin=0  OutMax=4  OutDataTypeStr=int8
  Cyber : Subsystem
  M{,1..3} (4 alike) : Memory
  Physical : Subsystem
  S1 : Subsystem
  S2 : Subsystem
  S3 : Subsystem
  S4 : Subsystem
  W1Pos : Outport
  W2Pos : Outport  Port=2
  W3Pos : Outport  Port=3
  W4Pos : Outport  Port=4
  wires:
  Cyber/4(W4) -> Physical/4(InW4)
  Physical/4(W4) -> S4/1(PhyMeasure), W4Pos/1
  DW2/1 -> Cyber/6(DW2)
  P3W4/1 -> Cyber/10(P3W4)
  S2/1(SensorOut) -> M1/1
  Physical/2(W2) -> S2/1(PhyMeasure), W2Pos/1
  DW1/1 -> Cyber/5(DW1)
  M/1 -> Cyber/1(PosW1)
  Physical/3(W3) -> S3/1(PhyMeasure), W3Pos/1
  M1/1 -> Cyber/2(PosW2)
  S4/1(SensorOut) -> M3/1
  DW3/1 -> Cyber/7(DW3)
  O3/1 -> Cyber/13(OW3)
  CW1C/1 -> Cyber/16(CW1C)
  P1W2/1 -> Cyber/8(P1W2)
  M2/1 -> Cyber/3(PosW3)
  Cyber/2(W2) -> Physical/2(InW2)
  Cyber/1(W1) -> Physical/1(InW1)
  O1/1 -> Cyber/11(OW1)
  LD/1 -> Cyber/15(LD)
  Cyber/3(W3) -> Physical/3(InW3)
  O2/1 -> Cyber/12(OW2)
  S3/1(SensorOut) -> M2/1
  O4/1 -> Cyber/14(OW4)
  Physical/1(W1) -> S1/1(PhyMeasure), W1Pos/1
  CW4C/1 -> Cyber/18(CW4C)
  CW2C/1 -> Cyber/17(CW2C)
  S1/1(SensorOut) -> M/1
  P2W3/1 -> Cyber/9(P2W3)
  M3/1 -> Cyber/4(PosW4)

== system c00007M_harness/M018 ==
  DW1 : Inport  OutMin=0  OutMax=4  OutDataTypeStr=int8
  DW2 : Inport  Port=2  OutMin=0  OutMax=4  OutDataTypeStr=int8
  DW3 : Inport  Port=3  OutMin=0  OutMax=4  OutDataTypeStr=int8
  P1W2 : Inport  Port=4  OutMin=0  OutMax=4  OutDataTypeStr=int8
  P2W3 : Inport  Port=5  OutMin=0  OutMax=4  OutDataTypeStr=int8
  P3W4 : Inport  Port=6  OutMin=0  OutMax=4  OutDataTypeStr=int8
  O1 : Inport  Port=7  OutDataTypeStr=boolean
  O2 : Inport  Port=8  OutDataTypeStr=boolean
  O3 : Inport  Port=9  OutDataTypeStr=boolean
  O4 : Inport  Port=10  OutDataTypeStr=boolean
  LD : Inport  Port=11  OutDataTypeStr=boolean
  CW1C : Inport  Port=12  OutMin=0  OutMax=4  OutDataTypeStr=int8
  CW2C : Inport  Port=13  OutMin=0  OutMax=4  OutDataTypeStr=int8
  CW4C : Inport  Port=14  OutMin=0  OutMax=4  OutDataTypeStr=int8
  Cyber : Subsystem
  M{,1..3} (4 alike) : Memory
  Physical : Subsystem
  S1 : Subsystem
  S2 : Subsystem
  S3 : Subsystem
  S4 : Subsystem
  W1Pos : Outport
  W2Pos : Outport  Port=2
  W3Pos : Outport  Port=3
  W4Pos : Outport  Port=4
  wires:
  Cyber/4(W4) -> Physical/4(InW4)
  Physical/4(W4) -> S4/1(PhyMeasure), W4Pos/1
  DW2/1 -> Cyber/6(DW2)
  P3W4/1 -> Cyber/10(P3W4)
  S2/1(SensorOut) -> M1/1
  Physical/2(W2) -> S2/1(PhyMeasure), W2Pos/1
  DW1/1 -> Cyber/5(DW1)
  M/1 -> Cyber/1(PosW1)
  Physical/3(W3) -> S3/1(PhyMeasure), W3Pos/1
  M1/1 -> Cyber/2(PosW2)
  S4/1(SensorOut) -> M3/1
  DW3/1 -> Cyber/7(DW3)
  O3/1 -> Cyber/13(OW3)
  CW1C/1 -> Cyber/16(CW1C)
  P1W2/1 -> Cyber/8(P1W2)
  M2/1 -> Cyber/3(PosW3)
  Cyber/2(W2) -> Physical/2(InW2)
  Cyber/1(W1) -> Physical/1(InW1)
  O1/1 -> Cyber/11(OW1)
  LD/1 -> Cyber/15(LD)
  Cyber/3(W3) -> Physical/3(InW3)
  O2/1 -> Cyber/12(OW2)
  S3/1(SensorOut) -> M2/1
  O4/1 -> Cyber/14(OW4)
  Physical/1(W1) -> S1/1(PhyMeasure), W1Pos/1
  CW4C/1 -> Cyber/18(CW4C)
  CW2C/1 -> Cyber/17(CW2C)
  S1/1(SensorOut) -> M/1
  P2W3/1 -> Cyber/9(P2W3)
  M3/1 -> Cyber/4(PosW4)

== system c00007M_harness/M019 ==
  DW1 : Inport  OutMin=0  OutMax=4  OutDataTypeStr=int8
  DW2 : Inport  Port=2  OutMin=0  OutMax=4  OutDataTypeStr=int8
  DW3 : Inport  Port=3  OutMin=0  OutMax=4  OutDataTypeStr=int8
  P1W2 : Inport  Port=4  OutMin=0  OutMax=4  OutDataTypeStr=int8
  P2W3 : Inport  Port=5  OutMin=0  OutMax=4  OutDataTypeStr=int8
  P3W4 : Inport  Port=6  OutMin=0  OutMax=4  OutDataTypeStr=int8
  O1 : Inport  Port=7  OutDataTypeStr=boolean
  O2 : Inport  Port=8  OutDataTypeStr=boolean
  O3 : Inport  Port=9  OutDataTypeStr=boolean
  O4 : Inport  Port=10  OutDataTypeStr=boolean
  LD : Inport  Port=11  OutDataTypeStr=boolean
  CW1C : Inport  Port=12  OutMin=0  OutMax=4  OutDataTypeStr=int8
  CW2C : Inport  Port=13  OutMin=0  OutMax=4  OutDataTypeStr=int8
  CW4C : Inport  Port=14  OutMin=0  OutMax=4  OutDataTypeStr=int8
  Cyber : Subsystem
  M{,1..3} (4 alike) : Memory
  Physical : Subsystem
  S1 : Subsystem
  S2 : Subsystem
  S3 : Subsystem
  S4 : Subsystem
  W1Pos : Outport
  W2Pos : Outport  Port=2
  W3Pos : Outport  Port=3
  W4Pos : Outport  Port=4
  wires:
  Cyber/4(W4) -> Physical/4(InW4)
  Physical/4(W4) -> S4/1(PhyMeasure), W4Pos/1
  DW2/1 -> Cyber/6(DW2)
  P3W4/1 -> Cyber/10(P3W4)
  S2/1(SensorOut) -> M1/1
  Physical/2(W2) -> S2/1(PhyMeasure), W2Pos/1
  DW1/1 -> Cyber/5(DW1)
  M/1 -> Cyber/1(PosW1)
  Physical/3(W3) -> S3/1(PhyMeasure), W3Pos/1
  M1/1 -> Cyber/2(PosW2)
  S4/1(SensorOut) -> M3/1
  DW3/1 -> Cyber/7(DW3)
  O3/1 -> Cyber/13(OW3)
  CW1C/1 -> Cyber/16(CW1C)
  P1W2/1 -> Cyber/8(P1W2)
  M2/1 -> Cyber/3(PosW3)
  Cyber/2(W2) -> Physical/2(InW2)
  Cyber/1(W1) -> Physical/1(InW1)
  O1/1 -> Cyber/11(OW1)
  LD/1 -> Cyber/15(LD)
  Cyber/3(W3) -> Physical/3(InW3)
  O2/1 -> Cyber/12(OW2)
  S3/1(SensorOut) -> M2/1
  O4/1 -> Cyber/14(OW4)
  Physical/1(W1) -> S1/1(PhyMeasure), W1Pos/1
  CW4C/1 -> Cyber/18(CW4C)
  CW2C/1 -> Cyber/17(CW2C)
  S1/1(SensorOut) -> M/1
  P2W3/1 -> Cyber/9(P2W3)
  M3/1 -> Cyber/4(PosW4)

== system c00007M_harness/M020 ==
  DW1 : Inport  OutMin=0  OutMax=4  OutDataTypeStr=int8
  DW2 : Inport  Port=2  OutMin=0  OutMax=4  OutDataTypeStr=int8
  DW3 : Inport  Port=3  OutMin=0  OutMax=4  OutDataTypeStr=int8
  P1W2 : Inport  Port=4  OutMin=0  OutMax=4  OutDataTypeStr=int8
  P2W3 : Inport  Port=5  OutMin=0  OutMax=4  OutDataTypeStr=int8
  P3W4 : Inport  Port=6  OutMin=0  OutMax=4  OutDataTypeStr=int8
  O1 : Inport  Port=7  OutDataTypeStr=boolean
  O2 : Inport  Port=8  OutDataTypeStr=boolean
  O3 : Inport  Port=9  OutDataTypeStr=boolean
  O4 : Inport  Port=10  OutDataTypeStr=boolean
  LD : Inport  Port=11  OutDataTypeStr=boolean
  CW1C : Inport  Port=12  OutMin=0  OutMax=4  OutDataTypeStr=int8
  CW2C : Inport  Port=13  OutMin=0  OutMax=4  OutDataTypeStr=int8
  CW4C : Inport  Port=14  OutMin=0  OutMax=4  OutDataTypeStr=int8
  Cyber : Subsystem
  M{,1..3} (4 alike) : Memory
  Physical : Subsystem
  S1 : Subsystem
  S2 : Subsystem
  S3 : Subsystem
  S4 : Subsystem
  W1Pos : Outport
  W2Pos : Outport  Port=2
  W3Pos : Outport  Port=3
  W4Pos : Outport  Port=4
  wires:
  Cyber/4(W4) -> Physical/4(InW4)
  Physical/4(W4) -> S4/1(PhyMeasure), W4Pos/1
  DW2/1 -> Cyber/6(DW2)
  P3W4/1 -> Cyber/10(P3W4)
  S2/1(SensorOut) -> M1/1
  Physical/2(W2) -> S2/1(PhyMeasure), W2Pos/1
  DW1/1 -> Cyber/5(DW1)
  M/1 -> Cyber/1(PosW1)
  Physical/3(W3) -> S3/1(PhyMeasure), W3Pos/1
  M1/1 -> Cyber/2(PosW2)
  S4/1(SensorOut) -> M3/1
  DW3/1 -> Cyber/7(DW3)
  O3/1 -> Cyber/13(OW3)
  CW1C/1 -> Cyber/16(CW1C)
  P1W2/1 -> Cyber/8(P1W2)
  M2/1 -> Cyber/3(PosW3)
  Cyber/2(W2) -> Physical/2(InW2)
  Cyber/1(W1) -> Physical/1(InW1)
  O1/1 -> Cyber/11(OW1)
  LD/1 -> Cyber/15(LD)
  Cyber/3(W3) -> Physical/3(InW3)
  O2/1 -> Cyber/12(OW2)
  S3/1(SensorOut) -> M2/1
  O4/1 -> Cyber/14(OW4)
  Physical/1(W1) -> S1/1(PhyMeasure), W1Pos/1
  CW4C/1 -> Cyber/18(CW4C)
  CW2C/1 -> Cyber/17(CW2C)
  S1/1(SensorOut) -> M/1
  P2W3/1 -> Cyber/9(P2W3)
  M3/1 -> Cyber/4(PosW4)
